simulink model "hydrophone"  (R2017a)
settings: Solver=FixedStepDiscrete  StartTime=0.0  StopTime=.1  RelTol=1e-3
undefined symbols (not defined in the file or in its folder): coefficients
libraries: simulink x10, dspxfrm3 x7, dspsrcs4 x4, dsphdlfiltering x4, dspmathops x3, hdlsllib x3
settings Model: MinMaxOverflowLogging=MinMaxAndOverflow  FPTRunName=NoOverride  SimulationMode=accelerator  PauseTimes=.03  NumberOfSteps=1000  Creator=jeffr  LastModifiedBy=jy4661
settings SolverCC: AutoInsertRateTranBlk=on
settings DataIOCC: LimitDataPoints=on  SaveOutput=off  SignalLogging=off  SaveTime=off
settings OptimizationCC: BlockReduction=off  ConditionallyExecuteInputs=off  DefaultParameterBehavior=Inlined  LifeSpan=inf
settings DebuggingCC: AlgebraicLoopMsg=error  SingleTaskRateTransMsg=error  AllowSymbolicDim=off  SFUnexpectedBacktrackingDiag=warning  SFNoUnconditionalDefaultTransitionDiag=warning  SFExecutionAtInitializationDiag=none
settings HardwareCC: ProdBitPerPointer=32  ProdBitPerSizeT=32  ProdBitPerPtrDiffT=32  ProdLargestAtomicFloat=None  ProdIntDivRoundTo=Undefined  ProdEndianess=Unspecified  ProdWordSize=32  ProdHWDeviceType=ASIC/FPGA->ASIC/FPGA  ProdEqTarget=off
settings GRTTargetCC: TargetLangStandard=C89/C90 (ANSI)  GeneratePreprocessorConditionals=Disable all
settings ConfigComp: CovMetricSettings=dw  CovHtmlReporting=on  CovSaveCumulativeToWorkspaceVar=on  CovSaveSingleToWorkspaceVar=on  CovExternalEMLEnable=off  CovSFcnEnable=off  DVTestSuiteOptimization=CombinedObjectives (Nonlinear Extended)  DVDetectFloatOverflow=off

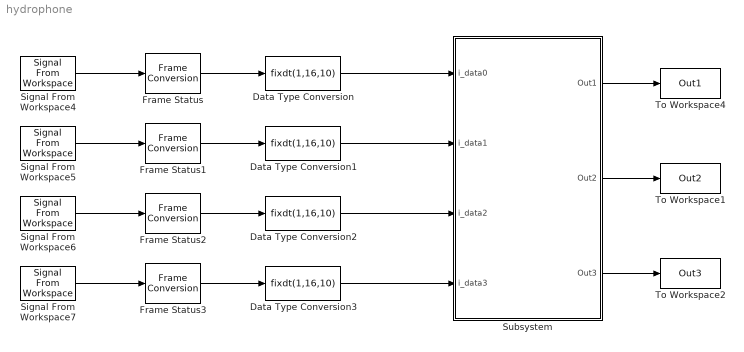
== system hydrophone ==
  Data Type Conversion{,1..3} (4 alike) : DataTypeConversion  OutDataTypeStr=fixdt(1,16,10)
  Frame Status{,1..3} (4 alike) : FrameConversion  InheritSamplingMode=off  OutFrame=Sample-based
  Signal From Workspace4 : dspsrcs4/Signal From Workspace  X=data0  Ts=1e-5  nsamps=1  OutputAfterFinalValue=Setting to zero  ignoreOrWarnInputAndFrameLengths=off  OutputFrames=off
  Signal From Workspace5 : dspsrcs4/Signal From Workspace  X=data1  Ts=1e-5  nsamps=1  OutputAfterFinalValue=Setting to zero  ignoreOrWarnInputAndFrameLengths=off  OutputFrames=off
  Signal From Workspace6 : dspsrcs4/Signal From Workspace  X=data1  Ts=1e-5  nsamps=1  OutputAfterFinalValue=Setting to zero  ignoreOrWarnInputAndFrameLengths=off  OutputFrames=off
  Signal From Workspace7 : dspsrcs4/Signal From Workspace  X=data1  Ts=1e-5  nsamps=1  OutputAfterFinalValue=Setting to zero  ignoreOrWarnInputAndFrameLengths=off  OutputFrames=off
  Subsystem : Subsystem  TreatAsAtomicUnit=on
  To Workspace1 : ToWorkspace  VariableName=Out2  SampleTime=-1
      settings: Save2DSignal=2-D array (concatenate along first dimension)
  To Workspace2 : ToWorkspace  VariableName=Out3  SampleTime=-1
      settings: Save2DSignal=2-D array (concatenate along first dimension)
  To Workspace4 : ToWorkspace  VariableName=Out1  SampleTime=-1
      settings: Save2DSignal=2-D array (concatenate along first dimension)
  wires:
  Signal From Workspace5/1 -> Frame Status1/1
  Signal From Workspace4/1 -> Frame Status/1
  Signal From Workspace6/1 -> Frame Status2/1
  Signal From Workspace7/1 -> Frame Status3/1
  Frame Status/1 -> Data Type Conversion/1
  Frame Status1/1 -> Data Type Conversion1/1
  Frame Status2/1 -> Data Type Conversion2/1
  Frame Status3/1 -> Data Type Conversion3/1
  Data Type Conversion/1 -> Subsystem/1(i_data0)
  Data Type Conversion1/1 -> Subsystem/2(i_data1)
  Data Type Conversion2/1 -> Subsystem/3(i_data2)
  Data Type Conversion3/1 -> Subsystem/4(i_data3)
  Subsystem/1(Out1) -> To Workspace4/1
  Subsystem/2(Out2) -> To Workspace1/1
  Subsystem/3(Out3) -> To Workspace2/1

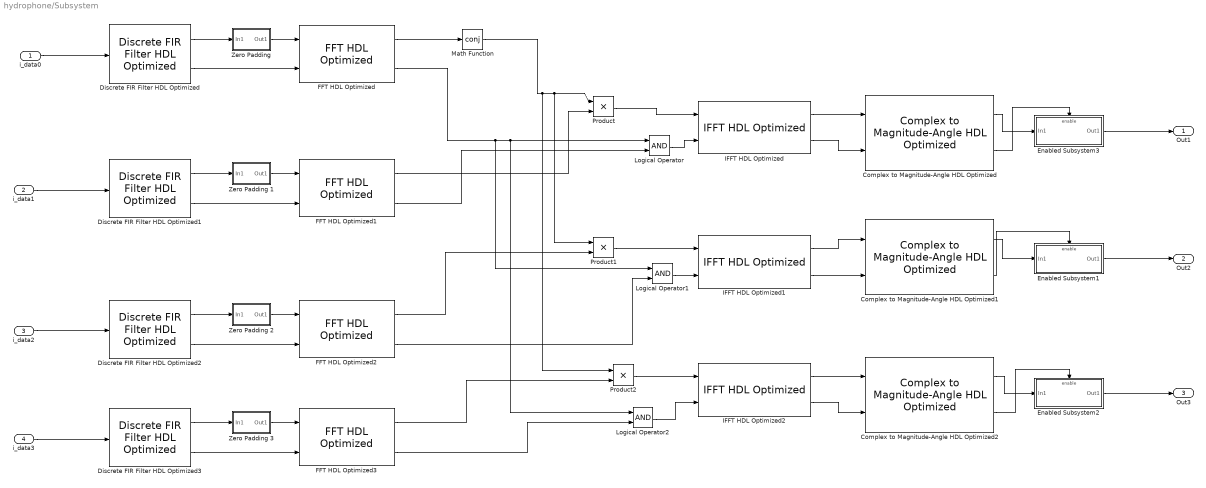
== system hydrophone/Subsystem ==
  i_data0 : Inport
  i_data1 : Inport  Port=2
  i_data2 : Inport  Port=3
  i_data3 : Inport  Port=4
  Complex to Magnitude-Angle HDL Optimized : dspmathops/Complex to Magnitude-Angle HDL Optimized  NumIterationsSource=Auto  NumIterations=10  OutputFormat=Magnitude  AngleFormat=Normalized  ScaleOutput=on  SimulateUsing=Code generation
      settings: SourceProductName=DSP System Toolbox  SourceProductBaseCode=DS
  Complex to Magnitude-Angle HDL Optimized1 : dspmathops/Complex to Magnitude-Angle HDL Optimized  NumIterationsSource=Auto  NumIterations=10  OutputFormat=Magnitude  AngleFormat=Normalized  ScaleOutput=on  SimulateUsing=Code generation
      settings: SourceProductName=DSP System Toolbox  SourceProductBaseCode=DS
  Complex to Magnitude-Angle HDL Optimized2 : dspmathops/Complex to Magnitude-Angle HDL Optimized  NumIterationsSource=Auto  NumIterations=10  OutputFormat=Magnitude  AngleFormat=Normalized  ScaleOutput=on  SimulateUsing=Code generation
      settings: SourceProductName=DSP System Toolbox  SourceProductBaseCode=DS
  Discrete FIR Filter HDL Optimized{,1..3} (4 alike) : dsphdlfiltering/Discrete FIR Filter HDL Optimized  Numerator=coefficients  Sharing=off  SharingFactor=2  SimulateUsing=Code generation  roundingMode=Floor  overflowMode=off  CoefficientsDataTypeStr=Inherit: Same word length as input  CoefficientsMin=[]  CoefficientsMax=[]  OutputDataTypeStr=Inherit: Same word length as input  OutputMin=[]  OutputMax=[]  ValidInPort=off  ReadyPort=off
      settings: SourceProductName=DSP System Toolbox  SourceProductBaseCode=DS
  Enabled Subsystem1 : Subsystem  TreatAsAtomicUnit=on
  Enabled Subsystem2 : Subsystem  TreatAsAtomicUnit=on
  Enabled Subsystem3 : Subsystem  TreatAsAtomicUnit=on
  FFT HDL Optimized{,1..3} (4 alike) : dspxfrm3/FFT HDL Optimized  FFTLength=512  Architecture=Streaming Radix 2^2  ComplexMultiplication=Use 3 multipliers and 5 adders  BitReversedOutput=off  BitReversedInput=off  Normalize=off  SimulateUsing=Code generation  RoundingMethod=Floor  ResetInputPort=off  StartOutputPort=off  EndOutputPort=off
      settings: SourceProductName=DSP System Toolbox  SourceProductBaseCode=DS
  IFFT HDL Optimized : dspxfrm3/IFFT HDL Optimized  FFTLength=512  Architecture=Streaming Radix 2^2  ComplexMultiplication=Use 3 multipliers and 5 adders  BitReversedOutput=off  BitReversedInput=off  Normalize=on  SimulateUsing=Code generation  RoundingMethod=Floor  ResetInputPort=off  StartOutputPort=off  EndOutputPort=off
      settings: SourceProductName=DSP System Toolbox  SourceProductBaseCode=DS
  IFFT HDL Optimized1 : dspxfrm3/IFFT HDL Optimized  FFTLength=512  Architecture=Streaming Radix 2^2  ComplexMultiplication=Use 3 multipliers and 5 adders  BitReversedOutput=off  BitReversedInput=off  Normalize=on  SimulateUsing=Code generation  RoundingMethod=Floor  ResetInputPort=off  StartOutputPort=off  EndOutputPort=off
      settings: SourceProductName=DSP System Toolbox  SourceProductBaseCode=DS
  IFFT HDL Optimized2 : dspxfrm3/IFFT HDL Optimized  FFTLength=512  Architecture=Streaming Radix 2^2  ComplexMultiplication=Use 3 multipliers and 5 adders  BitReversedOutput=off  BitReversedInput=off  Normalize=on  SimulateUsing=Code generation  RoundingMethod=Floor  ResetInputPort=off  StartOutputPort=off  EndOutputPort=off
      settings: SourceProductName=DSP System Toolbox  SourceProductBaseCode=DS
  Logical Operator : Logic  AllPortsSameDT=off  OutDataTypeStr=boolean
  Logical Operator1 : Logic  AllPortsSameDT=off  OutDataTypeStr=boolean
  Logical Operator2 : Logic  AllPortsSameDT=off  OutDataTypeStr=boolean
  Math Function : Math  Operator=conj  SaturateOnIntegerOverflow=on
  Product : Product
  Product1 : Product
  Product2 : Product
  "Zero Padding " : Subsystem
  Zero Padding 1 : Subsystem
  Zero Padding 2 : Subsystem
  Zero Padding 3 : Subsystem
  Out1 : Outport
  Out2 : Outport  Port=2
  Out3 : Outport  Port=3
  wires:
  FFT HDL Optimized/1 -> Math Function/1
  FFT HDL Optimized1/1 -> Product/2
  Logical Operator/1 -> IFFT HDL Optimized/2
  Math Function/1 -> Product2/1, Product1/1, Product/1
  FFT HDL Optimized1/2 -> Logical Operator/2
  FFT HDL Optimized/2 -> Logical Operator1/1, Logical Operator2/1, Logical Operator/1
  IFFT HDL Optimized/2 -> Complex to Magnitude-Angle HDL Optimized/2
  Discrete FIR Filter HDL Optimized2/2 -> FFT HDL Optimized2/2
  Logical Operator1/1 -> IFFT HDL Optimized1/2
  Logical Operator2/1 -> IFFT HDL Optimized2/2
  FFT HDL Optimized2/2 -> Logical Operator1/2
  FFT HDL Optimized3/2 -> Logical Operator2/2
  Product1/1 -> IFFT HDL Optimized1/1
  FFT HDL Optimized3/1 -> Product2/2
  FFT HDL Optimized2/1 -> Product1/2
  IFFT HDL Optimized1/1 -> Complex to Magnitude-Angle HDL Optimized1/1
  IFFT HDL Optimized1/2 -> Complex to Magnitude-Angle HDL Optimized1/2
  IFFT HDL Optimized2/1 -> Complex to Magnitude-Angle HDL Optimized2/1
  IFFT HDL Optimized2/2 -> Complex to Magnitude-Angle HDL Optimized2/2
  Product2/1 -> IFFT HDL Optimized2/1
  Complex to Magnitude-Angle HDL Optimized/2 -> Enabled Subsystem3/Enable
  Complex to Magnitude-Angle HDL Optimized/1 -> Enabled Subsystem3/1(In1)
  Product/1 -> IFFT HDL Optimized/1
  IFFT HDL Optimized/1 -> Complex to Magnitude-Angle HDL Optimized/1
  Enabled Subsystem3/1(Out1) -> Out1/1
  Enabled Subsystem1/1(Out1) -> Out2/1
  Complex to Magnitude-Angle HDL Optimized1/1 -> Enabled Subsystem1/1(In1)
  Complex to Magnitude-Angle HDL Optimized1/2 -> Enabled Subsystem1/Enable
  Enabled Subsystem2/1(Out1) -> Out3/1
  Complex to Magnitude-Angle HDL Optimized2/2 -> Enabled Subsystem2/Enable
  Complex to Magnitude-Angle HDL Optimized2/1 -> Enabled Subsystem2/1(In1)
  i_data0/1 -> Discrete FIR Filter HDL Optimized/1
  Discrete FIR Filter HDL Optimized/1 -> "Zero Padding "/1(In1)
  Discrete FIR Filter HDL Optimized/2 -> FFT HDL Optimized/2
  i_data1/1 -> Discrete FIR Filter HDL Optimized1/1
  Discrete FIR Filter HDL Optimized1/1 -> Zero Padding 1/1(In1)
  Discrete FIR Filter HDL Optimized1/2 -> FFT HDL Optimized1/2
  i_data2/1 -> Discrete FIR Filter HDL Optimized2/1
  Discrete FIR Filter HDL Optimized2/1 -> Zero Padding 2/1(In1)
  i_data3/1 -> Discrete FIR Filter HDL Optimized3/1
  Discrete FIR Filter HDL Optimized3/1 -> Zero Padding 3/1(In1)
  Discrete FIR Filter HDL Optimized3/2 -> FFT HDL Optimized3/2
  Zero Padding 3/1(Out1) -> FFT HDL Optimized3/1
  Zero Padding 2/1(Out1) -> FFT HDL Optimized2/1
  Zero Padding 1/1(Out1) -> FFT HDL Optimized1/1
  "Zero Padding "/1(Out1) -> FFT HDL Optimized/1

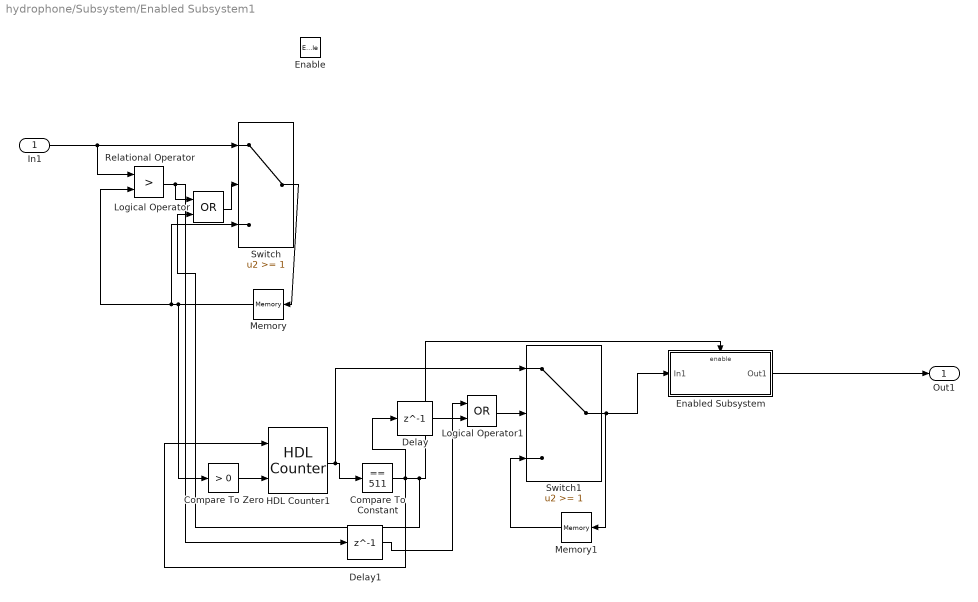
== system hydrophone/Subsystem/Enabled Subsystem1 ==
  In1 : Inport
  Enable : EnablePort  StatesWhenEnabling=reset
  Compare To Constant : simulink/Logic and Bit Operations/Compare To Constant  relop===  const=511  OutDataTypeStr=boolean
  Compare To Zero : simulink/Logic and Bit Operations/Compare To Zero  relop=>  OutDataTypeStr=boolean
  Delay : Delay  DelayLength=1  InitialCondition=0
  Delay1 : Delay  DelayLength=1  InitialCondition=0
  Enabled Subsystem : Subsystem  TreatAsAtomicUnit=on
  HDL Counter1 : hdlsllib/HDL Operations/HDL Counter  CountType=Count limited  CountInit=0  CountStep=1  CountMax=511  CountFromType=Specify  CountFrom=0  CountResetPort=on  CountLoadPort=off  CountEnbPort=on  CountDirPort=off  CountDataType=Signed  CountWordLen=10  CountFracLen=0  CountSampTime=1
      settings: SourceProductName=HDL Coder  SourceProductBaseCode=HD
  Logical Operator : Logic  Operator=OR  AllPortsSameDT=off  OutDataTypeStr=boolean
  Logical Operator1 : Logic  Operator=OR  AllPortsSameDT=off  OutDataTypeStr=boolean
  Memory : Memory  InheritSampleTime=on
  Memory1 : Memory  InheritSampleTime=on
  Relational Operator : RelationalOperator  Operator=>  OutDataTypeStr=boolean  RndMeth=Nearest
  Switch : Switch  Threshold=1
  Switch1 : Switch  Threshold=1
  Out1 : Outport  InitialOutput=0
  wires:
  Enabled Subsystem/1(Out1) -> Out1/1
  Delay1/1 -> Logical Operator1/1
  Delay/1 -> Logical Operator1/2
  Compare To Constant/1 -> Enabled Subsystem/Enable, Logical Operator/2, HDL Counter1/1, Delay/1
  HDL Counter1/1 -> Compare To Constant/1, Switch1/1
  Logical Operator1/1 -> Switch1/2
  Memory1/1 -> Switch1/3
  Switch1/1 -> Enabled Subsystem/1(In1), Memory1/1
  Logical Operator/1 -> Switch/2
  Compare To Zero/1 -> HDL Counter1/2
  Relational Operator/1 -> Logical Operator/1, Delay1/1
  In1/1 -> Relational Operator/1, Switch/1
  Memory/1 -> Switch/3, Relational Operator/2, Compare To Zero/1
  Switch/1 -> Memory/1

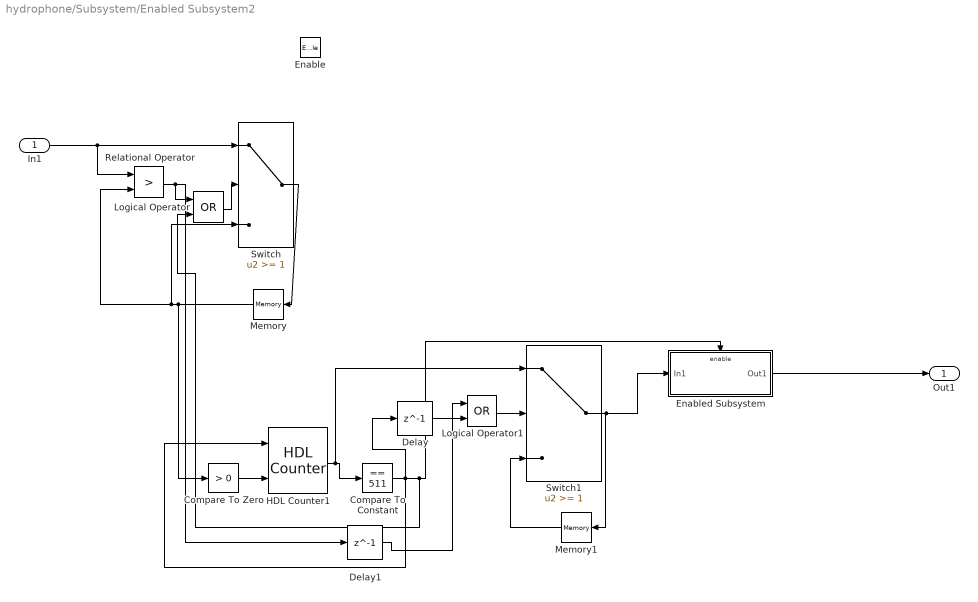
== system hydrophone/Subsystem/Enabled Subsystem2 ==
  In1 : Inport
  Enable : EnablePort  StatesWhenEnabling=reset
  Compare To Constant : simulink/Logic and Bit Operations/Compare To Constant  relop===  const=511  OutDataTypeStr=boolean
  Compare To Zero : simulink/Logic and Bit Operations/Compare To Zero  relop=>  OutDataTypeStr=boolean
  Delay : Delay  DelayLength=1  InitialCondition=0
  Delay1 : Delay  DelayLength=1  InitialCondition=0
  Enabled Subsystem : Subsystem  TreatAsAtomicUnit=on
  HDL Counter1 : hdlsllib/HDL Operations/HDL Counter  CountType=Count limited  CountInit=0  CountStep=1  CountMax=511  CountFromType=Specify  CountFrom=0  CountResetPort=on  CountLoadPort=off  CountEnbPort=on  CountDirPort=off  CountDataType=Signed  CountWordLen=10  CountFracLen=0  CountSampTime=1
      settings: SourceProductName=HDL Coder  SourceProductBaseCode=HD
  Logical Operator : Logic  Operator=OR  AllPortsSameDT=off  OutDataTypeStr=boolean
  Logical Operator1 : Logic  Operator=OR  AllPortsSameDT=off  OutDataTypeStr=boolean
  Memory : Memory  InheritSampleTime=on
  Memory1 : Memory  InheritSampleTime=on
  Relational Operator : RelationalOperator  Operator=>  OutDataTypeStr=boolean  RndMeth=Nearest
  Switch : Switch  Threshold=1
  Switch1 : Switch  Threshold=1
  Out1 : Outport  InitialOutput=0
  wires:
  Switch/1 -> Memory/1
  Memory/1 -> Compare To Zero/1, Relational Operator/2, Switch/3
  In1/1 -> Switch/1, Relational Operator/1
  Relational Operator/1 -> Delay1/1, Logical Operator/1
  Compare To Zero/1 -> HDL Counter1/2
  Logical Operator/1 -> Switch/2
  Switch1/1 -> Memory1/1, Enabled Subsystem/1(In1)
  Memory1/1 -> Switch1/3
  Logical Operator1/1 -> Switch1/2
  HDL Counter1/1 -> Switch1/1, Compare To Constant/1
  Compare To Constant/1 -> Delay/1, HDL Counter1/1, Logical Operator/2, Enabled Subsystem/Enable
  Delay/1 -> Logical Operator1/2
  Delay1/1 -> Logical Operator1/1
  Enabled Subsystem/1(Out1) -> Out1/1

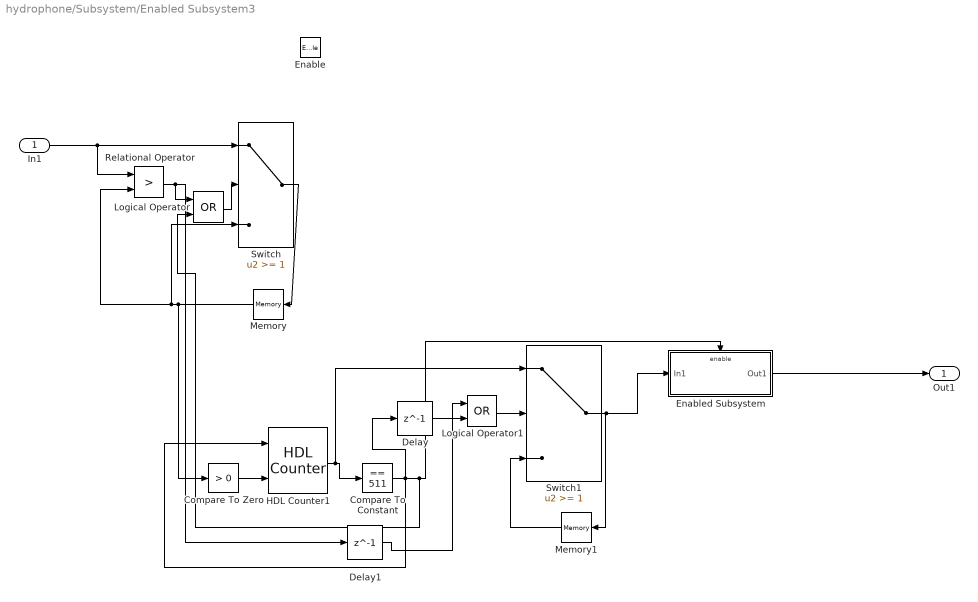
== system hydrophone/Subsystem/Enabled Subsystem3 ==
  In1 : Inport
  Enable : EnablePort  StatesWhenEnabling=reset
  Compare To Constant : simulink/Logic and Bit Operations/Compare To Constant  relop===  const=511  OutDataTypeStr=boolean
  Compare To Zero : simulink/Logic and Bit Operations/Compare To Zero  relop=>  OutDataTypeStr=boolean
  Delay : Delay  DelayLength=1  InitialCondition=0
  Delay1 : Delay  DelayLength=1  InitialCondition=0
  Enabled Subsystem : Subsystem  TreatAsAtomicUnit=on
  HDL Counter1 : hdlsllib/HDL Operations/HDL Counter  CountType=Count limited  CountInit=0  CountStep=1  CountMax=511  CountFromType=Specify  CountFrom=0  CountResetPort=on  CountLoadPort=off  CountEnbPort=on  CountDirPort=off  CountDataType=Signed  CountWordLen=10  CountFracLen=0  CountSampTime=1
      settings: SourceProductName=HDL Coder  SourceProductBaseCode=HD
  Logical Operator : Logic  Operator=OR  AllPortsSameDT=off  OutDataTypeStr=boolean
  Logical Operator1 : Logic  Operator=OR  AllPortsSameDT=off  OutDataTypeStr=boolean
  Memory : Memory  InheritSampleTime=on
  Memory1 : Memory  InheritSampleTime=on
  Relational Operator : RelationalOperator  Operator=>  OutDataTypeStr=boolean  RndMeth=Nearest
  Switch : Switch  Threshold=1
  Switch1 : Switch  Threshold=1
  Out1 : Outport  InitialOutput=0
  wires:
  Switch/1 -> Memory/1
  Memory/1 -> Compare To Zero/1, Relational Operator/2, Switch/3
  In1/1 -> Switch/1, Relational Operator/1
  Relational Operator/1 -> Delay1/1, Logical Operator/1
  Compare To Zero/1 -> HDL Counter1/2
  Logical Operator/1 -> Switch/2
  Switch1/1 -> Memory1/1, Enabled Subsystem/1(In1)
  Memory1/1 -> Switch1/3
  Logical Operator1/1 -> Switch1/2
  HDL Counter1/1 -> Switch1/1, Compare To Constant/1
  Compare To Constant/1 -> Delay/1, HDL Counter1/1, Logical Operator/2, Enabled Subsystem/Enable
  Delay/1 -> Logical Operator1/2
  Delay1/1 -> Logical Operator1/1
  Enabled Subsystem/1(Out1) -> Out1/1

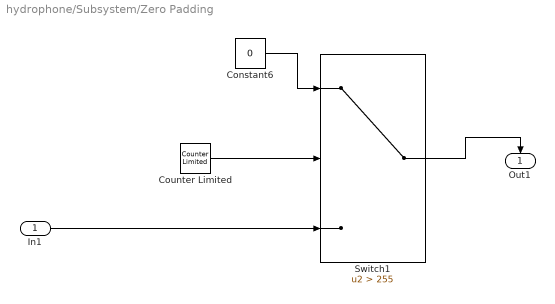
== system hydrophone/Subsystem/Zero Padding  ==
  In1 : Inport
  Constant6 : Constant  Value=0  OutDataTypeStr=uint8
  Counter Limited : simulink/Sources/Counter Limited  uplimit=7  tsamp=-1
  Switch1 : Switch  Criteria=u2 > Threshold  Threshold=255
  Out1 : Outport
  wires:
  Constant6/1 -> Switch1/1
  In1/1 -> Switch1/3
  Switch1/1 -> Out1/1
  Counter Limited/1 -> Switch1/2

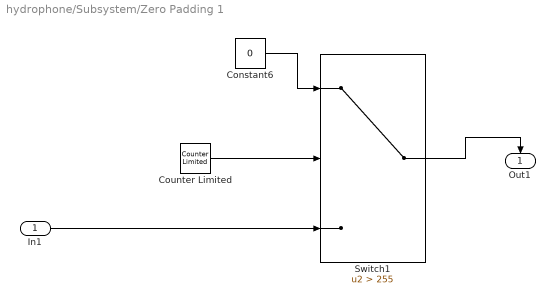
== system hydrophone/Subsystem/Zero Padding 1 ==
  In1 : Inport
  Constant6 : Constant  Value=0  OutDataTypeStr=uint8
  Counter Limited : simulink/Sources/Counter Limited  uplimit=7  tsamp=-1
  Switch1 : Switch  Criteria=u2 > Threshold  Threshold=255
  Out1 : Outport
  wires:
  Counter Limited/1 -> Switch1/2
  Switch1/1 -> Out1/1
  In1/1 -> Switch1/3
  Constant6/1 -> Switch1/1

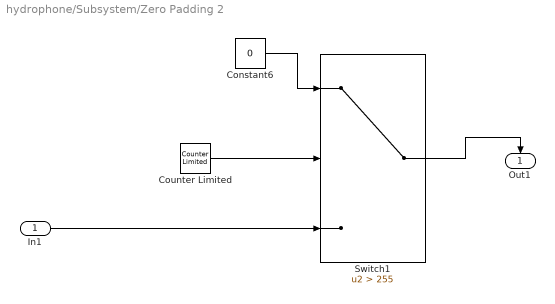
== system hydrophone/Subsystem/Zero Padding 2 ==
  In1 : Inport
  Constant6 : Constant  Value=0  OutDataTypeStr=uint8
  Counter Limited : simulink/Sources/Counter Limited  uplimit=7  tsamp=-1
  Switch1 : Switch  Criteria=u2 > Threshold  Threshold=255
  Out1 : Outport
  wires:
  Constant6/1 -> Switch1/1
  In1/1 -> Switch1/3
  Switch1/1 -> Out1/1
  Counter Limited/1 -> Switch1/2

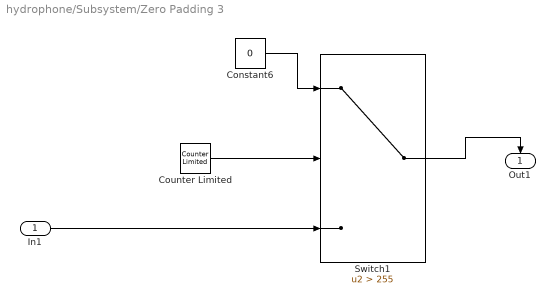
== system hydrophone/Subsystem/Zero Padding 3 ==
  In1 : Inport
  Constant6 : Constant  Value=0  OutDataTypeStr=uint8
  Counter Limited : simulink/Sources/Counter Limited  uplimit=7  tsamp=-1
  Switch1 : Switch  Criteria=u2 > Threshold  Threshold=255
  Out1 : Outport
  wires:
  Counter Limited/1 -> Switch1/2
  Switch1/1 -> Out1/1
  In1/1 -> Switch1/3
  Constant6/1 -> Switch1/1

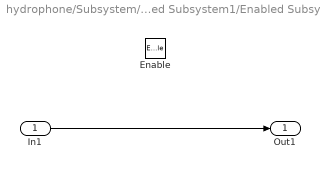
== system hydrophone/Subsystem/Enabled Subsystem1/Enabled Subsystem ==
  In1 : Inport
  Enable : EnablePort  StatesWhenEnabling=reset
  Out1 : Outport  OutputWhenDisabled=reset  InitialOutput=0
  wires:
  In1/1 -> Out1/1

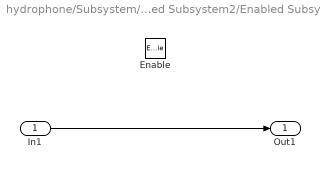
== system hydrophone/Subsystem/Enabled Subsystem2/Enabled Subsystem ==
  In1 : Inport
  Enable : EnablePort  StatesWhenEnabling=reset
  Out1 : Outport  OutputWhenDisabled=reset  InitialOutput=0
  wires:
  In1/1 -> Out1/1

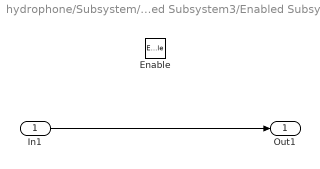
== system hydrophone/Subsystem/Enabled Subsystem3/Enabled Subsystem ==
  In1 : Inport
  Enable : EnablePort  StatesWhenEnabling=reset
  Out1 : Outport  OutputWhenDisabled=reset  InitialOutput=0
  wires:
  In1/1 -> Out1/1
